simulink model "clik_control"  (R2019a)
settings: Solver=FixedStepAuto  StartTime=0.0  StopTime=inf  FixedStep=0.001  RelTol=1e-3
undefined symbols (not defined in the file or in its folder): Force
libraries: robotlib x5, simulink x2, eeGeneralControl x2
settings Model: Creator=huic  LastModifiedBy=huic

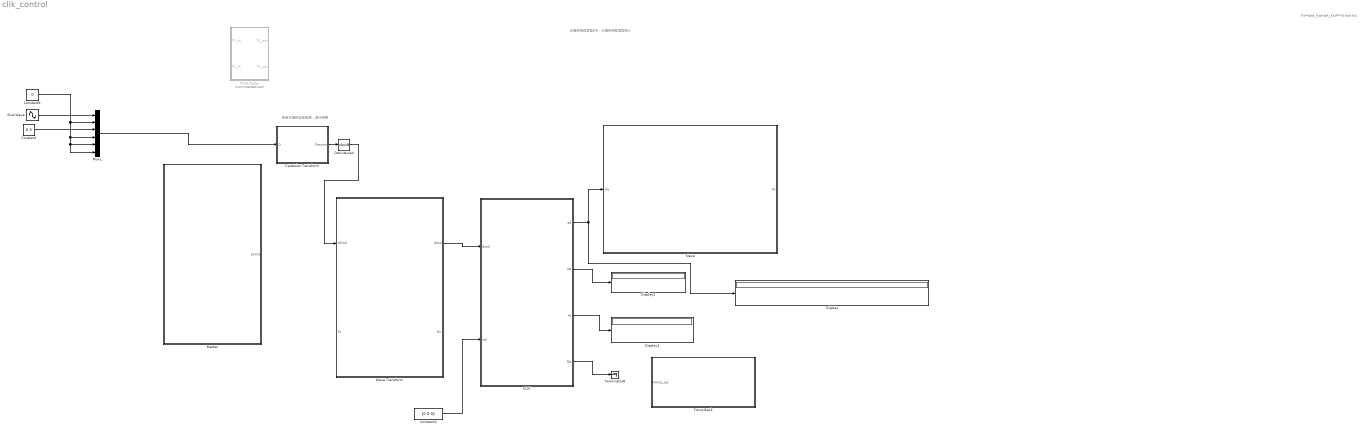
== system clik_control ==
  note: FS=(dot_Xsd-dot_Xs)*P+I(Xsd-Xs)
  note: 来自主端的位姿信息，进行映射
  note: 主端采用改进型DH，从端采用标准型DH
  " Time Delay" : Subsystem  Commented=on
  CLIK : Subsystem
  Cartesian Transform : MATLAB Function  TreatAsAtomicUnit=on
  Constant : Constant  Value=0.3
  Constant2 : Constant  Value=[0 0 0]'
  Constant6 : Constant  Value=0
  Derivative4 : Derivative
  Display : Display
  Display1 : Display
  Display2 : Display
  Force Back : Subsystem
  Master : Subsystem
  Mux1 : Mux  Inputs=6
  Sine Wave : Sin  Amplitude=0.8  Frequency=0.5  SampleTime=0
  Slave : Subsystem
  Terminator8 : Terminator
  Wave Transform : Subsystem
  wires:
  CLIK/2(we) -> Display2/1
  CLIK/3(xe) -> Display1/1
  Constant2/1 -> CLIK/2(wd)
  CLIK/4(Dp) -> Terminator8/1
  Constant6/1 -> Mux1/6, Mux1/5, Mux1/4, Mux1/2
  Constant/1 -> Mux1/3
  Sine Wave/1 -> Mux1/1
  Cartesian Transform/1(Postion) -> Derivative4/1
  CLIK/1(qd) -> Display/1, Slave/1(dq)
  Wave Transform/1(dXsd) -> CLIK/1(dxsd)
  Mux1/1 -> Cartesian Transform/1(Q)
  Derivative4/1 -> Wave Transform/1(dXmd)

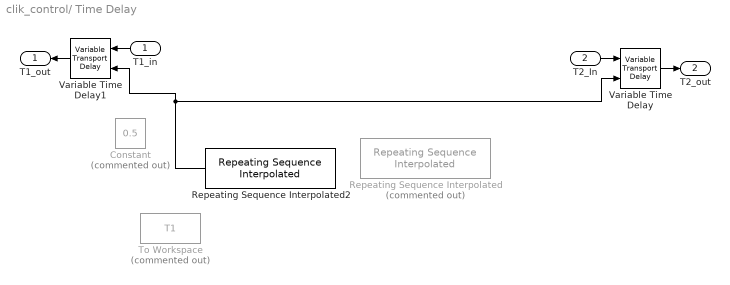
== system clik_control/ Time Delay ==
  T1_in : Inport
  T2_In : Inport  Port=2
  Constant : Constant  Commented=on  Value=0.5
  Repeating Sequence Interpolated : simulink/Sources/Repeating Sequence Interpolated  Commented=on  OutValues=[0 0 0.21 0.23 0.03 0.03 0.215 0.235 0.03].'  TimeValues=[0 2 4 8 10 12 14 18 20].'  LookUpMeth=Interpolation-Use End Values  tsamp=0.01  OutMin=[]  OutMax=[]  OutDataTypeStr=double  OutputDataTypeScalingMode=double  OutDataType=fixdt(0,8)  OutScaling=2^-10
  Repeating Sequence Interpolated2 : simulink/Sources/Repeating Sequence Interpolated  OutValues=[0 0 0.8 0.82 0.03 0].'  TimeValues=[0 2 4 8 9.8 10].'  LookUpMeth=Interpolation-Use End Values  tsamp=0.01  OutMin=[]  OutMax=[]  OutDataTypeStr=double  OutputDataTypeScalingMode=double  OutDataType=fixdt(0,8)  OutScaling=2^-10
  To Workspace : ToWorkspace  Commented=on  VariableName=T1  SaveFormat=Structure With Time  SampleTime=-1
  Variable Time Delay : VariableTransportDelay  MaximumDelay=10  MaximumPoints=10240  ZeroDelay=on
  Variable Time Delay1 : VariableTransportDelay  MaximumDelay=10  MaximumPoints=10240  ZeroDelay=on
  T1_out : Outport
  T2_out : Outport  Port=2
  wires:
  T1_in/1 -> Variable Time Delay1/1
  Variable Time Delay1/1 -> T1_out/1
  Variable Time Delay/1 -> T2_out/1
  T2_In/1 -> Variable Time Delay/1
  Repeating Sequence Interpolated2/1 -> Variable Time Delay1/2, Variable Time Delay/2

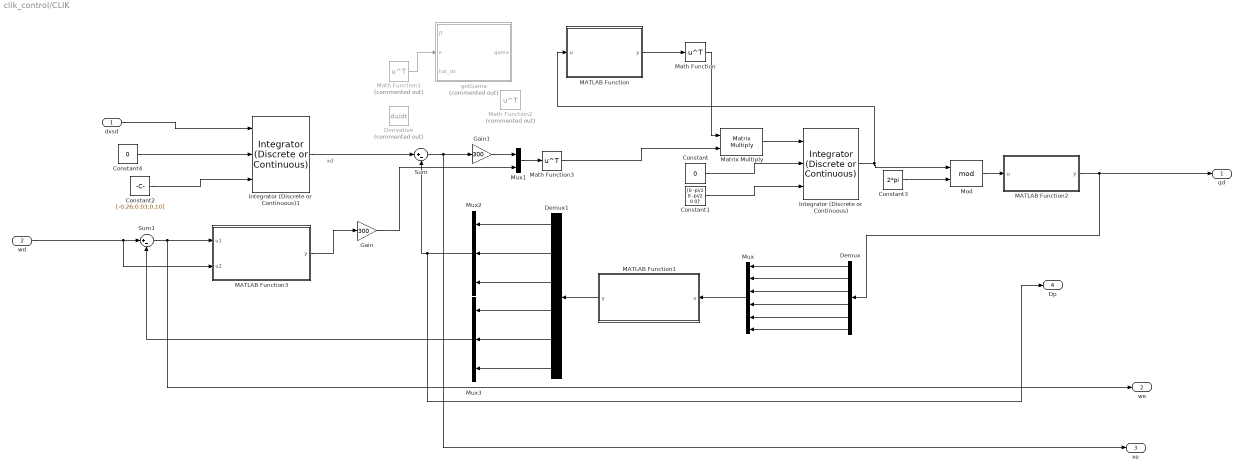
== system clik_control/CLIK ==
  note: xd
  dxsd : Inport
  wd : Inport  Port=2
  Constant : Constant  Value=0
  Constant1 : Constant  Value=[0 -pi/2 0 -pi/2 0 0]'
  Constant2 : Constant  Value=[-0.26;0.03;0.10]
  Constant3 : Constant  Value=2*pi
  Constant4 : Constant  Value=0
  Demux : Demux  Outputs=[1 1 1 1 1 1]
  Demux1 : Demux  Outputs=[1 1 1 1 1 1]
  Derivative : Derivative  Commented=on
  Gain : Gain  Gain=300
  Gain1 : Gain  Gain=300
  Integrator (Discrete or Continuous) : eeGeneralControl/Integrator (Discrete or Continuous)  LabelModeActiveChoice=Continuous  ExternalReset=level  LimitType=Anti-windup  B=inf  A=-inf  Ts=0
      settings: SourceProductName=Simscape Electrical  SourceProductBaseCode=PS
  Integrator (Discrete or Continuous)1 : eeGeneralControl/Integrator (Discrete or Continuous)  LabelModeActiveChoice=Discrete  ExternalReset=level  LimitType=Anti-windup  B=[0.45;0.45;0.55]  A=[-0.45;-0.45;-0.12]  Ts=-1
      settings: SourceProductName=Simscape Electrical  SourceProductBaseCode=PS
  MATLAB Function : MATLAB Function  TreatAsAtomicUnit=on
  MATLAB Function1 : MATLAB Function  TreatAsAtomicUnit=on
  MATLAB Function2 : MATLAB Function  TreatAsAtomicUnit=on
  MATLAB Function3 : MATLAB Function  TreatAsAtomicUnit=on
  Math Function : Math  Operator=transpose  SaturateOnIntegerOverflow=on
  Math Function1 : Math  Commented=on  Operator=transpose  SaturateOnIntegerOverflow=on
  Math Function2 : Math  Commented=on  Operator=transpose  SaturateOnIntegerOverflow=on
  Math Function3 : Math  Operator=transpose  SaturateOnIntegerOverflow=on
  Matrix Multiply : Product  Multiplication=Matrix(*)
  Mod : Math  Operator=mod  SaturateOnIntegerOverflow=on
  Mux : Mux  Inputs=[1 1 1 1 1 1]
  Mux1 : Mux  Inputs=2
  Mux2 : Mux  Inputs=[1 1 1]
  Mux3 : Mux  Inputs=[1 1 1]
  Sum : Sum  Inputs=|+-
  Sum1 : Sum  Inputs=|+-
  getGama : MATLAB Function  Commented=on  TreatAsAtomicUnit=on
  qd : Outport
  we : Outport  Port=2
  xe : Outport  Port=3
  Dp : Outport  Port=4
  wires:
  Demux/2 -> Mux/2
  Integrator (Discrete or Continuous)/1 -> MATLAB Function/1(u), Mod/1
  Math Function/1 -> Matrix Multiply/1
  Demux/5 -> Mux/5
  Mux/1 -> MATLAB Function1/1(u)
  MATLAB Function2/1(y) -> qd/1, Demux/1
  Demux/4 -> Mux/4
  Demux1/5 -> Mux3/2
  Demux/6 -> Mux/6
  wd/1 -> MATLAB Function3/2(u2), Sum1/1
  Demux/1 -> Mux/1
  Demux/3 -> Mux/3
  Matrix Multiply/1 -> Integrator (Discrete or Continuous)/1
  Mux3/1 -> Sum1/2
  Constant3/1 -> Mod/2
  Mux2/1 -> Sum/2, Dp/1
  Demux1/4 -> Mux3/1
  Mod/1 -> MATLAB Function2/1(u)
  Demux1/1 -> Mux2/1
  Demux1/2 -> Mux2/2
  MATLAB Function1/1(y) -> Demux1/1
  Demux1/3 -> Mux2/3
  Sum1/1 -> we/1, MATLAB Function3/1(u1)
  Constant1/1 -> Integrator (Discrete or Continuous)/3
  Demux1/6 -> Mux3/3
  Constant/1 -> Integrator (Discrete or Continuous)/2
  MATLAB Function/1(y) -> Math Function/1
  Constant4/1 -> Integrator (Discrete or Continuous)1/2
  dxsd/1 -> Integrator (Discrete or Continuous)1/1
  Constant2/1 -> Integrator (Discrete or Continuous)1/3
  Sum/1 -> Gain1/1, xe/1
  Math Function3/1 -> Matrix Multiply/2
  Integrator (Discrete or Continuous)1/1 -> Sum/1
  Math Function1/1 -> getGama/2(e)
  MATLAB Function3/1(y) -> Gain/1
  Gain1/1 -> Mux1/1
  Gain/1 -> Mux1/2
  Mux1/1 -> Math Function3/1

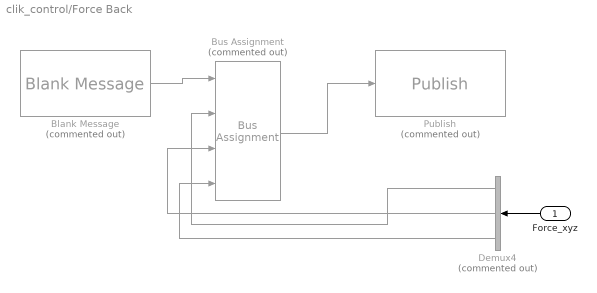
== system clik_control/Force Back ==
  Force_xyz : Inport
  Blank Message : robotlib/Blank Message  Commented=on  messageClass=Message  entityType=omni_msgs/OmniFeedback  messageType=omni_msgs/OmniFeedback  SampleTime=inf
      settings: SourceProductBaseCode=RO
  Bus Assignment : BusAssignment  Commented=on  AssignedSignals=Force.X,Force.Y,Force.Z
  Demux4 : Demux  Commented=on  Outputs=3
  Publish : robotlib/Publish  Commented=on  topicSource=Select from ROS network  topic=/phantom/phantom/force_feedback  messageType=omni_msgs/OmniFeedback  messageQueueLength=1
      settings: SourceProductBaseCode=RO
  wires:
  Demux4/3 -> Bus Assignment/4
  Demux4/2 -> Bus Assignment/3
  Bus Assignment/1 -> Publish/1
  Blank Message/1 -> Bus Assignment/1
  Force_xyz/1 -> Demux4/1
  Demux4/1 -> Bus Assignment/2

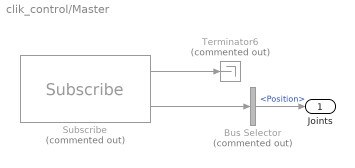
== system clik_control/Master ==
  Bus Selector : BusSelector  Commented=on  OutputSignals=Position
  Subscribe : robotlib/Subscribe  Commented=on  topicSource=Select from ROS network  topic=/phantom/phantom/joint_states  messageType=sensor_msgs/JointState  sampleTime=-1  messageQueueLength=1
      settings: SourceProductBaseCode=RO
  Terminator6 : Terminator  Commented=on
  Joints : Outport
  wires:
  Bus Selector/1 -> Joints/1  "<Position>"
  Subscribe/1 -> Terminator6/1
  Subscribe/2 -> Bus Selector/1

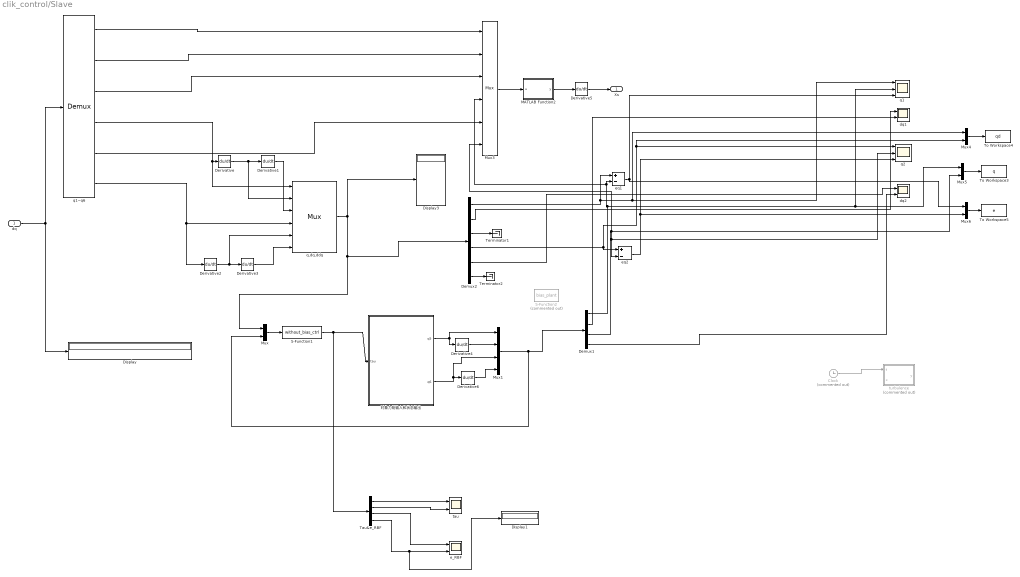
== system clik_control/Slave ==
  dq : Inport
  Clock : Clock  Commented=on
  Demux1 : Demux
  Demux2 : Demux  Outputs=6
  Derivative{,1..6} (7 alike) : Derivative
  Display : Display
  Display1 : Display
  Display3 : Display
  MATLAB Function2 : MATLAB Function  TreatAsAtomicUnit=on
  Mux{,4..6} (4 alike) : Mux  Inputs=2
  Mux1 : Mux
  Mux3 : Mux  Inputs=6
  S-Function1 : S-Function  FunctionName=without_bias_ctrl  SFunctionDeploymentMode=off  EnableBusSupport=off
  S-Function2 : S-Function  Commented=on  FunctionName=bias_plant  SFunctionDeploymentMode=off  EnableBusSupport=off
  Tau&e_RBF : Demux
  Terminator1 : Terminator
  Terminator2 : Terminator
  To Workspace3 : ToWorkspace  VariableName=q  SaveFormat=Structure With Time  SampleTime=-1
  To Workspace4 : ToWorkspace  VariableName=qd  SaveFormat=Structure With Time  SampleTime=-1
  To Workspace5 : ToWorkspace  VariableName=e  SaveFormat=Structure With Time  SampleTime=-1
  dq1 : Scope  NumInputPorts=2
  dq2 : Scope  NumInputPorts=2
  e_RBF : Scope  NumInputPorts=2
  eq1 : Sum  Inputs=+-
  eq2 : Sum  Inputs=+-
  q,dq,ddq : Mux  Inputs=6
  q1 : Scope  NumInputPorts=3
  q1~q6 : Demux  Outputs=6
  q2 : Scope  NumInputPorts=3
  tau : Scope  NumInputPorts=2
  turbulence : MATLAB Function  Commented=on  TreatAsAtomicUnit=on
  对象力矩输入和状态输出 : Subsystem
  Xs : Outport
  wires:
  Demux2/2 -> dq1/1
  Mux6/1 -> To Workspace5/1
  q1~q6/6 -> Derivative2/1, q,dq,ddq/4
  q1~q6/5 -> Mux3/5
  Tau&e_RBF/3 -> e_RBF/1
  dq/1 -> Display/1, q1~q6/1
  q,dq,ddq/1 -> Display3/1, Demux2/1, Mux/1
  S-Function1/1 -> Tau&e_RBF/1, 对象力矩输入和状态输出/1(tau)
  Demux1/3 -> Mux5/2, eq2/2, q2/2, Mux3/6
  Demux1/1 -> Mux3/4, eq1/2, Mux5/1, q1/2
  q1~q6/4 -> Derivative/1, q,dq,ddq/1
  eq2/1 -> Mux6/2, q2/3
  Clock/1 -> turbulence/1(t)
  Derivative5/1 -> Xs/1
  Derivative/1 -> Derivative1/1, q,dq,ddq/2
  Derivative2/1 -> Derivative3/1, q,dq,ddq/5
  q1~q6/2 -> Mux3/2
  Derivative1/1 -> q,dq,ddq/3
  Mux4/1 -> To Workspace4/1
  Demux2/3 -> Terminator1/1
  Demux2/6 -> Terminator2/1
  Demux1/4 -> dq2/2
  MATLAB Function2/1(y) -> Derivative5/1
  Demux2/4 -> Mux4/2, q2/1, eq2/1
  q1~q6/3 -> Mux3/3
  Derivative3/1 -> q,dq,ddq/6
  Mux3/1 -> MATLAB Function2/1(u)
  Tau&e_RBF/1 -> tau/1
  Demux2/5 -> dq2/1
  Tau&e_RBF/4 -> Display1/1, e_RBF/2
  Mux5/1 -> To Workspace3/1
  Mux/1 -> S-Function1/1
  q1~q6/1 -> Mux3/1
  Demux2/1 -> eq1/1, Mux4/1, q1/1
  Tau&e_RBF/2 -> tau/2
  eq1/1 -> Mux6/1, q1/3
  Demux1/2 -> dq1/2
  对象力矩输入和状态输出/1(q5) -> Mux1/1, Derivative4/1
  Derivative4/1 -> Mux1/2
  对象力矩输入和状态输出/2(q6) -> Mux1/3, Derivative6/1
  Derivative6/1 -> Mux1/4
  Mux1/1 -> Mux/2, Demux1/1

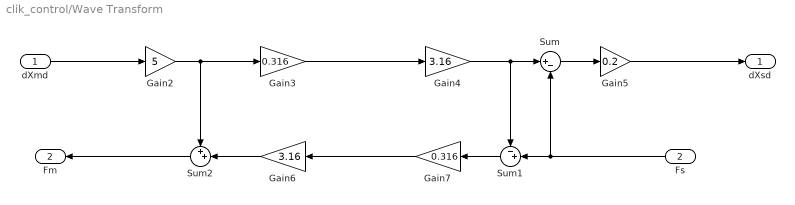
== system clik_control/Wave Transform ==
  dXmd : Inport
  Fs : Inport  Port=2
  Gain2 : Gain  Gain=5
  Gain3 : Gain  Gain=0.316
  Gain4 : Gain  Gain=3.16
  Gain5 : Gain  Gain=0.2
  Gain6 : Gain  Gain=3.16
  Gain7 : Gain  Gain=0.316
  Sum : Sum  Inputs=|+-
  Sum1 : Sum  Inputs=-+|
  Sum2 : Sum  Inputs=++|
  dXsd : Outport
  Fm : Outport  Port=2
  wires:
  Gain6/1 -> Sum2/2
  Gain2/1 -> Gain3/1, Sum2/1
  Sum2/1 -> Fm/1
  Gain3/1 -> Gain4/1
  Fs/1 -> Sum/2, Sum1/2
  Sum/1 -> Gain5/1
  Gain7/1 -> Gain6/1
  Sum1/1 -> Gain7/1
  Gain4/1 -> Sum1/1, Sum/1
  dXmd/1 -> Gain2/1
  Gain5/1 -> dXsd/1

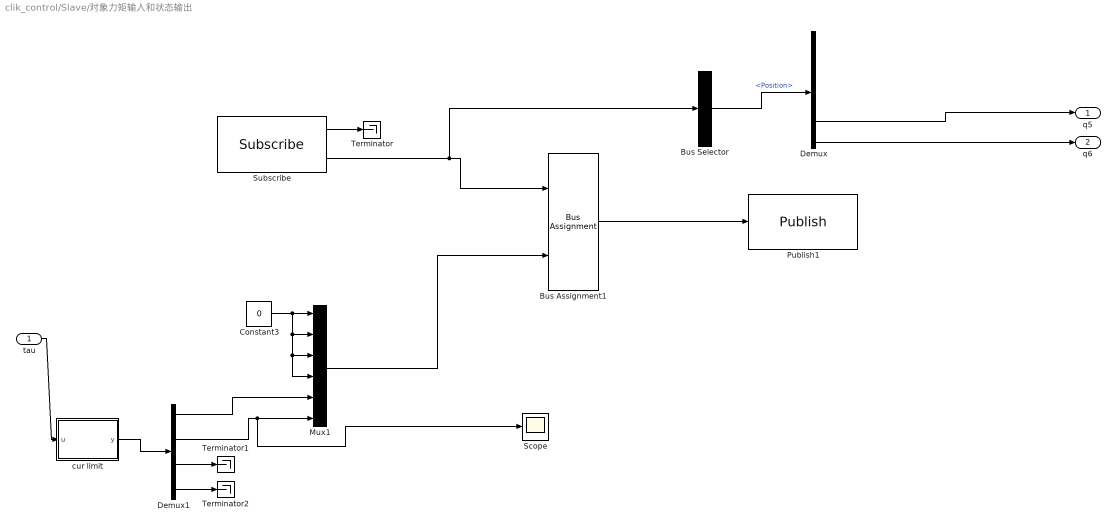
== system clik_control/Slave/对象力矩输入和状态输出 ==
  tau : Inport
  Bus Assignment1 : BusAssignment  AssignedSignals=Position
  Bus Selector : BusSelector  OutputSignals=Position
  Constant3 : Constant  Value=0
  Demux : Demux  Outputs=6
  Demux1 : Demux
  Mux1 : Mux  Inputs=6
  Publish1 : robotlib/Publish  topicSource=Select from ROS network  topic=/joint_states  messageType=sensor_msgs/JointState  messageQueueLength=1
      settings: SourceProductBaseCode=RO
  Scope : Scope
  Subscribe : robotlib/Subscribe  topicSource=Select from ROS network  topic=/joint_posStates  messageType=sensor_msgs/JointState  sampleTime=-1  messageQueueLength=1
      settings: SourceProductBaseCode=RO
  Terminator : Terminator
  Terminator1 : Terminator
  Terminator2 : Terminator
  cur limit : MATLAB Function  TreatAsAtomicUnit=on
  q5 : Outport
  q6 : Outport  Port=2
  wires:
  Demux/6 -> q6/1
  Bus Selector/1 -> Demux/1  "<Position>"
  Constant3/1 -> Mux1/4, Mux1/3, Mux1/2, Mux1/1
  Subscribe/1 -> Terminator/1
  Mux1/1 -> Bus Assignment1/2
  Bus Assignment1/1 -> Publish1/1
  Subscribe/2 -> Bus Selector/1, Bus Assignment1/1
  Demux/5 -> q5/1
  Demux1/1 -> Mux1/5
  Demux1/2 -> Scope/1, Mux1/6
  Demux1/3 -> Terminator1/1
  Demux1/4 -> Terminator2/1
  cur limit/1(y) -> Demux1/1
  tau/1 -> cur limit/1(u)

== matlab function clik_control/CLIK/MATLAB Function1 ==
  data: u input; y output
function y = getpose(u)
a2=-0.2035;a3=-0.17442;d1=0.1205;d4=0.08009;
d5=0.08009;
q1=u(1);
q2=u(2);
q3=u(3);
q4=u(4);
q5=u(5);
q6=u(6);
%求运动学正解
T01 = [cos(q1) 0 sin(q1) 0;sin(q1) 0 -cos(q1) 0;0 1 0 d1;0 0 0 1];
T12 = [cos(q2) -sin(q2) 0 a2*cos(q2);sin(q2) cos(q2) 0 a2*sin(q2);0 0 1 0;0 0 0 1];
T23 = [cos(q3) -sin(q3) 0 a3*cos(q3);sin(q3) cos(q3) 0 a3*sin(q3);0 0 1 0;0 0 0 1];
T34 = [cos(q4) 0 sin(q4) 0;sin(q4) 0 -cos(q4) 0;0 1 0 d4;0 0 0 1];
T45 = [cos(q5) 0 -sin(q5)  0;sin(q5) 0 cos(q5) 0;0 -1 0 d5;0 0 0 1];
T56 = [cos(q6) -sin(q6) 0 0;sin(q6) cos(q6) 0 0;0 0 1 0;0 0 0 1];
T06 = T01*T12*T23*T34*T45*T56;

y1=T06(1:3,4);
y2=tform2eul(T06);
y=[y1;y2'];

== matlab function clik_control/CLIK/MATLAB Function ==
  data: u input; y output
function y = getjacob(u)
%标准型雅可比矩阵求解
a2=-0.2035;a3=-0.17442;d1=0.1205;d4=0.08009;
d5=0.08009;
q=u;
%求运动学正解
T01 = [cos(q(1)) 0 sin(q(1)) 0;sin(q(1)) 0 -cos(q(1)) 0;0 1 0 d1;0 0 0 1];
T12 = [cos(q(2)) -sin(q(2)) 0 a2*cos(q(2));sin(q(2)) cos(q(2)) 0 a2*sin(q(2));0 0 1 0;0 0 0 1];
T23 = [cos(q(3)) -sin(q(3)) 0 a3*cos(q(3));sin(q(3)) cos(q(3)) 0 a3*sin(q(3));0 0 1 0;0 0 0 1];
T34 = [cos(q(4)) 0 sin(q(4)) 0;sin(q(4)) 0 -cos(q(4)) 0;0 1 0 d4;0 0 0 1];
T45 = [cos(q(5)) 0 -sin(q(5))  0;sin(q(5)) 0 cos(q(5)) 0;0 -1 0 d5;0 0 0 1];
T56 = [cos(q(6)) -sin(q(6)) 0 0;sin(q(6)) cos(q(6)) 0 0;0 0 1 0;0 0 0 1];

k = [0; 0; 1];

%初始赋值
Jv = zeros(3, 6);
Jw = zeros(3, 6);
%获取每个关节原点与基座标的变换矩阵T01,T02...T06
% T{6}=zeros(4);
T=cell(6,1);
T{1}=T01;
T{2}=T{1}*T12;
T{3}=T{2}*T23;
T{4}=T{3}*T34;
T{5}=T{4}*T45;
T{6}=T{5}*T56;

%进行矢量积求解
for i = 1: 6
   if i == 1
       R = eye(3);
       p_im = T{6}(1: 3, 4);
   else
       R = T{i-1}(1: 3, 1: 3);
       p_im = T{6}(1: 3, 4) - T{i-1}(1: 3, 4);
   end
   
   zi_1 = R * k;
   Jv(:, i) = cross(zi_1, p_im);
   Jw(:, i) = zi_1;
end

% 组合
J = [Jv; Jw];
y=J;

== matlab function clik_control/CLIK/MATLAB Function2 ==
  data: u input; y output
function y = Joints_angle_Handle(u)
for i=1:5
    if(u(i) > pi)
        u(i) = u(i)-2*pi;
    elseif(u(i) < -pi)
        u(i) = u(i)+2*pi;
    end
end
%限位
for i = 1 :5
    if(i == 2)
        if u(2) >1.75
            u(2) = 1.7;
        elseif u(2) < -1.75
            u(2) = -1.7;
        end
    else
        if u(i) >2.44
            u(i) = 2.4;
        elseif u(i) < -2.44
            u(i) = -2.4;
        end
    end
end
y = u;

== matlab function clik_control/CLIK/MATLAB Function3 ==
  data: u1 input; y output; u2 input
function y = anglevelocity(u1,u2)
%u2为当前的欧拉角
%u1为欧拉角的变化量
tform=[cos(u2(2))*cos(u2(3)) -sin(u2(3)) 0;cos(u2(2))*sin(u2(3)) cos(u2(3)) 0;-sin(u2(2)) 0 1];
y=zeros(1,3);
dwxyz=tform*[u1(3);u1(2);u1(1)];
y(1)=dwxyz(1);
y(2)=dwxyz(2);
y(3)=dwxyz(3);

== matlab function clik_control/Slave/turbulence ==
  data: t input; y output; x input
function y = turbulence(t,x)
Td=zeros(4,1);
if t>30&&t<35
    l1 = 0.35;  %unit is 'm'
    l2 = 0.31;  % li is the length of ith link i
    J=[-l1*sin(x(1))+l2*sin(x(1)+x(3))  -l2*sin(x(1)+x(3));  l1*cos(x(1))+l2*cos(x(1)+x(3))  l2*cos(x(1)+x(3)) ];
%     Td(1:2,:)=J'*[4,8]';
    Td(1:2,:)=J'*[10,16]';
end
y=Td;
end

== matlab function clik_control/Cartesian Transform ==
  data: Q input; Postion output
function Postion = TouchX_to_Gluon(Q)
d4=0.13335;d6=0.03;a2=0.13335;
q1=Q(1);q2=Q(2);q3=Q(3);q4=Q(4);q5=Q(5);q6=Q(6);
T01=[cos(q1) -sin(q1) 0 0;sin(q1) cos(q1) 0 0;0 0 1 0;0 0 0 1];
T12=[cos(q2) -sin(q2) 0 0;0 0 -1 0;sin(q2) cos(q2) 0 0;0 0 0 1];
T23=[cos(q3) -sin(q3) 0 a2;sin(q3) cos(q3) 0 0;0 0 1 0;0 0 0 1];
T34=[cos(q4) -sin(q4) 0 0;0 0 -1 -d4;sin(q4) cos(q4) 0 0;0 0 0 1];
T45=[cos(q5) -sin(q5) 0 0;0 0 -1 0;sin(q5) cos(q5) 0 0;0 0 0 1];
T56=[cos(q6) -sin(q6) 0 0;0 0 1 d6;-sin(q6) -cos(q6) 0 0;0 0 0 1];

% T06=T01*T12*T23*T34*T45*T56;

T06=T01*T12*T23*T34;
%进行映射转换
 Xg = 2.4*T06(1,4)-0.26;
 Yg = 1.8*T06(2,4)+0.03;
 Zg = 1.7*T06(3,4)+0.10;
  if Xg > -0.05 && Xg <= 0 && Yg > -0.05 && Yg < 0.05
    Xg= -0.05;
 elseif Xg < 0.05 && Xg >=0  && Yg > -0.05 && Yg < 0.05
        Xg = 0.05;
 end
%进行映射后的笛卡尔空间位置
P=[Xg;Yg;Zg];
% pose=tform2eul(T06);
Postion = P;
% Pose=pose';

== matlab function clik_control/Slave/MATLAB Function2 ==
  data: u input; y output
function y = Position(u)
a2=-0.2035;a3=-0.17442;d1=0.1205;d4=0.08009;
d5=0.08009;
q1=u(1);
q2=u(2);
q3=u(3);
q4=u(4);
q5=u(5);
q6=u(6);
%求运动学正解
T01 = [cos(q1) 0 sin(q1) 0;sin(q1) 0 -cos(q1) 0;0 1 0 d1;0 0 0 1];
T12 = [cos(q2) -sin(q2) 0 a2*cos(q2);sin(q2) cos(q2) 0 a2*sin(q2);0 0 1 0;0 0 0 1];
T23 = [cos(q3) -sin(q3) 0 a3*cos(q3);sin(q3) cos(q3) 0 a3*sin(q3);0 0 1 0;0 0 0 1];
T34 = [cos(q4) 0 sin(q4) 0;sin(q4) 0 -cos(q4) 0;0 1 0 d4;0 0 0 1];
T45 = [cos(q5) 0 -sin(q5)  0;sin(q5) 0 cos(q5) 0;0 -1 0 d5;0 0 0 1];
T56 = [cos(q6) -sin(q6) 0 0;sin(q6) cos(q6) 0 0;0 0 1 0;0 0 0 1];
T06 = T01*T12*T23*T34*T45*T56;

y1=T06(1:3,4);
y=y1;

== matlab function clik_control/CLIK/getGama ==
  data: JT input; gama output; e input; hat_dx input
function gama = SgetGama(JT,e,hat_dx)
alpha = 300;
res=zeros(6,6);
res(1,1)=alpha + (e'*hat_dx)/(e'*(JT'*JT)*e);
res(2,2)=alpha + (e'*hat_dx)/(e'*(JT'*JT)*e);
res(3,3)=alpha + (e'*hat_dx)/(e'*(JT'*JT)*e);
res(4,4)=alpha + (e'*hat_dx)/(e'*(JT'*JT)*e);
res(5,5)=alpha + (e'*hat_dx)/(e'*(JT'*JT)*e);
res(6,6)=alpha + (e'*hat_dx)/(e'*(JT'*JT)*e);
gama = res;

== matlab function clik_control/Slave/对象力矩输入和状态输出/cur limit ==
  data: u input; y output
function y = cur_limit(u)
if(u(2) > 2)
    u(2) = 2;
elseif (u(2) < -2)
    u(2) = -2;
end
y = u;
